simulink model "tune_launcher"  (R2018b)
settings: Solver=VariableStepAuto  StartTime=0.0  StopTime=10.0  RelTol=1e-3
settings Model: Creator=12819  LastModifiedBy=12819

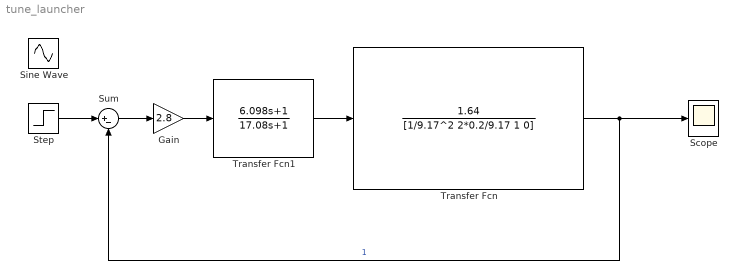
== system tune_launcher ==
  Gain : Gain  Gain=2.8
  Scope : Scope
  Sine Wave : Sin  Frequency=10  SampleTime=0
  Step : Step  Time=0  SampleTime=0
  Sum : Sum  Inputs=|+-
  Transfer Fcn : TransferFcn  Numerator=[1.64]  Denominator=[1/9.17^2 2*0.2/9.17 1 0]
  Transfer Fcn1 : TransferFcn  Numerator=[6.098 1]  Denominator=[17.08 1]
  wires:
  Transfer Fcn/1 -> Scope/1, Sum/2  "1"
  Sum/1 -> Gain/1
  Gain/1 -> Transfer Fcn1/1
  Transfer Fcn1/1 -> Transfer Fcn/1
  Step/1 -> Sum/1
